simulink model "H8_2GDL_partelinealizada"  (R2022b)
settings: Solver=VariableStepAuto  StartTime=0.0  StopTime=5  RelTol=1e-3
InitFcn:
  | load("hems.mat");
  | airgap = hems.Airgap;
  | current = hems.Current;
  | forceV = hems.Force_Vertical;
  | forceH = hems.Force_Horizontal;
  | inductance = hems.Inductance;
  | resistance = hems.Resistance;
  | 
  | m = 200;
  | g = 9.81;
  | Iyy = 26.887;
  | x_lev12 = 0.443;
  | x_lev34 = 0.542;
  | z_max = 0.0225;
  | z_min = 0.01;
  | z_nom = 0.01965;
  | I_max = 50;
  | I_min = -50;
settings Model: Creator=USUARIO  LastModifiedBy=aceao

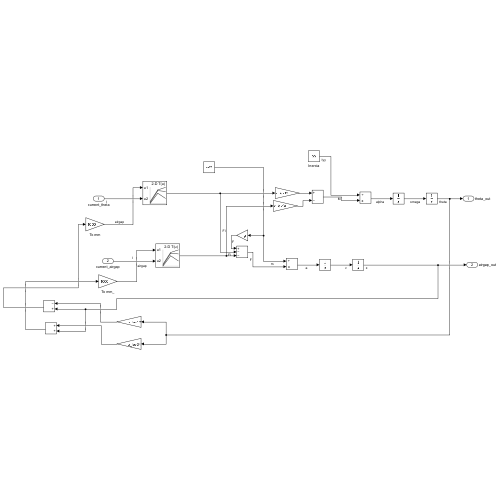
[thumbnail: Simulink's stored preview of the top-level diagram]
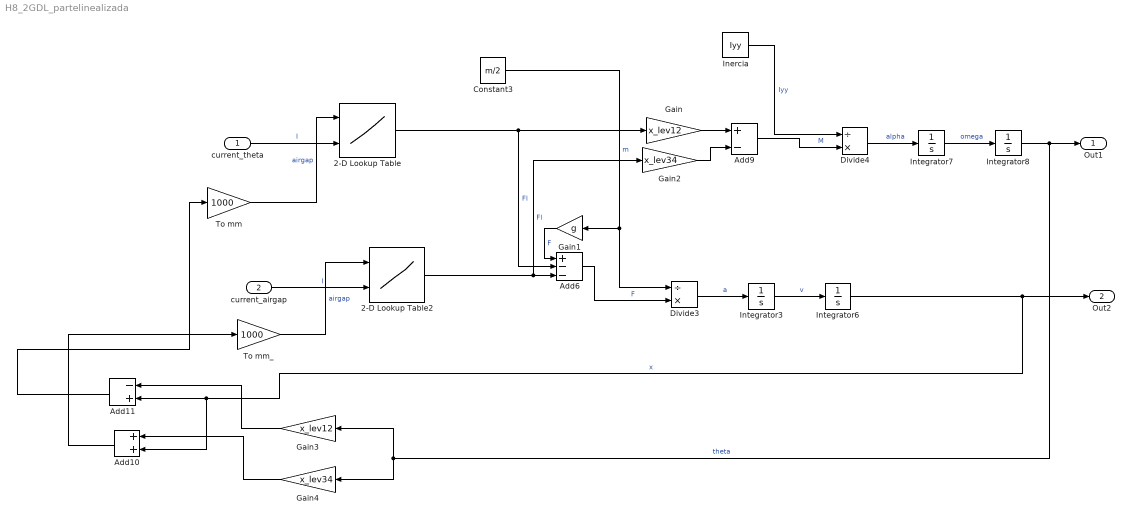
== system H8_2GDL_partelinealizada ==
  current_theta : Inport
  current_airgap : Inport  Port=2
  2-D Lookup Table : Lookup_n-D  BreakpointsForDimension1=airgap'  BreakpointsForDimension2=current  Table=forceV  InternalRulePriority=Speed  RndMeth=Simplest
      settings: InputPortMap=u0,u1
  2-D Lookup Table2 : Lookup_n-D  BreakpointsForDimension1=airgap'  BreakpointsForDimension2=current  Table=forceV  InternalRulePriority=Speed  RndMeth=Simplest
      settings: InputPortMap=u0,u1
  Add10 : Sum
  Add11 : Sum  Inputs=-+
  Add6 : Sum  Inputs=+--
  Add9 : Sum  Inputs=+-
  Constant3 : Constant  Value=m/2
  Divide3 : Product  Inputs=/*
  Divide4 : Product  Inputs=/*
  Gain : Gain  Gain=x_lev12
  Gain1 : Gain  Gain=g
  Gain2 : Gain  Gain=x_lev34
  Gain3 : Gain  Gain=x_lev12
  Gain4 : Gain  Gain=x_lev34
  Inercia : Constant  Value=Iyy
  Integrator3 : Integrator
  Integrator6 : Integrator  InitialCondition=z_nom
  Integrator7 : Integrator
  Integrator8 : Integrator
  To mm : Gain  Gain=1000
  To mm_ : Gain  Gain=1000
  Out1 : Outport  SignalName=theta_out
  Out2 : Outport  Port=2  SignalName=airgap_out
  wires:
  Integrator3/1 -> Integrator6/1  "v"
  To mm_/1 -> 2-D Lookup Table2/1  "airgap"
  Constant3/1 -> Gain1/1, Divide3/1  "m"
  Divide3/1 -> Integrator3/1  "a"
  2-D Lookup Table2/1 -> Gain2/1, Add6/3  "Fl"
  Integrator6/1 -> Out2/1, Add11/2, Add10/2  "x"
  Add6/1 -> Divide3/2  "F"
  current_airgap/1 -> 2-D Lookup Table2/2  "I"
  current_theta/1 -> 2-D Lookup Table/2  "I"
  To mm/1 -> 2-D Lookup Table/1  "airgap"
  2-D Lookup Table/1 -> Gain/1, Add6/2  "Fl"
  Add9/1 -> Divide4/2  "M"
  Integrator8/1 -> Out1/1, Gain4/1, Gain3/1  "theta"
  Divide4/1 -> Integrator7/1  "alpha"
  Integrator7/1 -> Integrator8/1  "omega"
  Inercia/1 -> Divide4/1  "Iyy"
  Add10/1 -> To mm_/1
  Add11/1 -> To mm/1
  Gain1/1 -> Add6/1  "F"
  Gain2/1 -> Add9/2
  Gain/1 -> Add9/1
  Gain3/1 -> Add11/1
  Gain4/1 -> Add10/1
